simulink model "OBserver_WithLQG_Control_Yaw"  (R2016a)
settings: Solver=VariableStepAuto  StartTime=0.0  StopTime=10.0  RelTol=1e-3
values from neighbouring files (symbols this model uses):
  denWd = [1 3.25]    [4OBserver_WithLQG_Control_structure_main.m]    (also in 5OBserver_WithLQG_Control_structure_tail.m = [1 0.20])
  denWn = [1 500.8]    [4OBserver_WithLQG_Control_structure_main.m]    (also in 5OBserver_WithLQG_Control_structure_tail.m = [1 800.8])
  Krt = lqr(A,B,Q,R)    [3LQG_for_TRAS_Yaw_angle.m]
  numWd = [3.25]    [4OBserver_WithLQG_Control_structure_main.m]    (also in 5OBserver_WithLQG_Control_structure_tail.m = [0.20])
  numWn = [1 0]    [4OBserver_WithLQG_Control_structure_main.m]    (also in 5OBserver_WithLQG_Control_structure_tail.m)
undefined symbols (not defined in the file or in its folder): at, bt, ct, dt, Ket
settings Model: Creator=engrh  LastModifiedBy=engrh

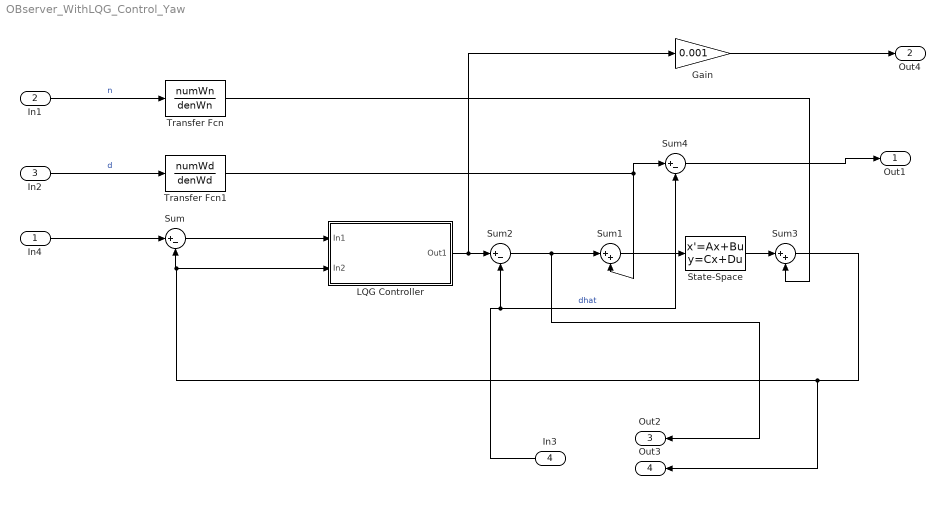
== system OBserver_WithLQG_Control_Yaw ==
  In4 : Inport
  In1 : Inport  Port=2
  In2 : Inport  Port=3
  In3 : Inport  Port=4
  Gain : Gain  Gain=0.001
  LQG Controller : Subsystem
  State-Space : StateSpace  A=at  B=bt  C=ct  D=dt  X0=0
  Sum : Sum  Inputs=|+-
  Sum1 : Sum  Inputs=|++
  Sum2 : Sum  Inputs=|+-
  Sum3 : Sum  Inputs=|++
  Sum4 : Sum  Inputs=|+-
  Transfer Fcn : TransferFcn  Numerator=numWn  Denominator=denWn
  Transfer Fcn1 : TransferFcn  Numerator=numWd  Denominator=denWd
  Out1 : Outport
  Out4 : Outport  Port=2
  Out2 : Outport  Port=3
  Out3 : Outport  Port=4
  wires:
  State-Space/1 -> Sum3/1
  Sum3/1 -> Out3/1, Sum/2, LQG Controller/2(In2)
  Sum/1 -> LQG Controller/1(In1)
  In1/1 -> Transfer Fcn/1  "n"
  Transfer Fcn/1 -> Sum3/2
  Sum1/1 -> State-Space/1
  LQG Controller/1(Out1) -> Gain/1, Sum2/1
  In2/1 -> Transfer Fcn1/1  "d"
  Transfer Fcn1/1 -> Sum4/1, Sum1/2
  In3/1 -> Sum4/2, Sum2/2  "dhat"
  Sum4/1 -> Out1/1
  Sum2/1 -> Out2/1, Sum1/1
  In4/1 -> Sum/1
  Gain/1 -> Out4/1

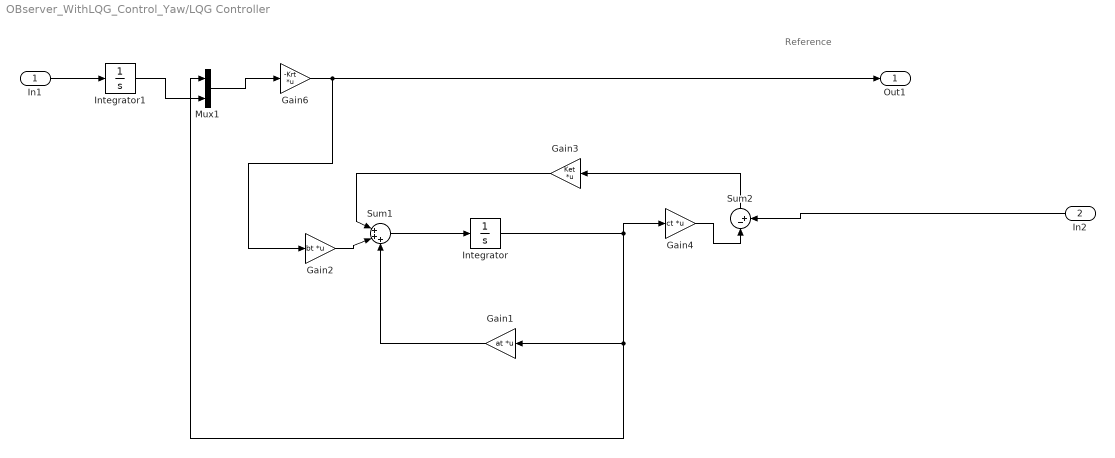
== system OBserver_WithLQG_Control_Yaw/LQG Controller ==
  note: Reference
  In1 : Inport
  In2 : Inport  Port=2
  Gain1 : Gain  Gain=at  Multiplication=Matrix(K*u)
  Gain2 : Gain  Gain=bt  Multiplication=Matrix(K*u)
  Gain3 : Gain  Gain=Ket  Multiplication=Matrix(K*u)
  Gain4 : Gain  Gain=ct  Multiplication=Matrix(K*u)
  Gain6 : Gain  Gain=-Krt  Multiplication=Matrix(K*u)
  Integrator : Integrator
  Integrator1 : Integrator
  Mux1 : Mux  Inputs=2
  Sum1 : Sum  Inputs=|+++
  Sum2 : Sum  Inputs=|-+
  Out1 : Outport
  wires:
  Mux1/1 -> Gain6/1
  Sum2/1 -> Gain3/1
  Gain4/1 -> Sum2/1
  Gain1/1 -> Sum1/3
  Sum1/1 -> Integrator/1
  Integrator/1 -> Mux1/1, Gain1/1, Gain4/1
  In1/1 -> Integrator1/1
  Integrator1/1 -> Mux1/2
  Gain6/1 -> Out1/1, Gain2/1
  Gain3/1 -> Sum1/1
  Gain2/1 -> Sum1/2
  In2/1 -> Sum2/2
